simulink model "Ctrl_WT_openPI_delay"  (R2019b)
settings: Solver=ode23tb  StartTime=0.0  StopTime=30  MaxStep=1/60  RelTol=1e-4  AbsTol=1e-3  EnableMultiTasking=on
InitFcn:
  | xInitial = init_power_wind_ig;
libraries: cstblocks x7
settings Model: PauseTimes=15  ExtModeAutoUpdateStatusClock=off  Creator=MathWorks  LastModifiedBy=estuser04
settings SolverCC: AutoScaleAbsTol=off  SolverResetMethod=Robust
settings DataIOCC: LimitDataPoints=on  SaveFormat=Array  SignalLoggingSaveFormat=ModelDataLogs  SaveOutput=off  SaveTime=off  ReturnWorkspaceOutputs=off  SignalLoggingName=logsOut
settings OptimizationCC: BlockReduction=off  DefaultParameterBehavior=Inlined  BufferReuse=off  ExpressionDepthLimit=2147483647  InitFltsAndDblsToZero=on  LifeSpan=inf
settings DebuggingCC: UnderspecifiedInitializationDetection=Classic  MergeDetectMultiDrivingBlocksExec=none  CheckExecutionContextPreStartOutputMsg=on  CheckExecutionContextRuntimeOutputMsg=on  SignalResolutionControl=TryResolveAllWithWarning  SolverPrmCheckMsg=warning  MultiTaskDSMMsg=warning  MultiTaskCondExecSysMsg=none  FcnCallInpInsideContextMsg=warning  StateNameClashWarn=warning  InitInArrayFormatMsg=none  SFUnexpectedBacktrackingDiag=warning  SFNoUnconditionalDefaultTransitionDiag=warning  SFExecutionAtInitializationDiag=none  ArithmeticOperatorsInVariantConditions=warning
settings HardwareCC: ProdBitPerPointer=32  ProdBitPerSizeT=32  ProdBitPerPtrDiffT=32  ProdLargestAtomicFloat=None  ProdIntDivRoundTo=Undefined  ProdEndianess=Unspecified  ProdWordSize=32  ProdHWDeviceType=32-bit Generic
settings ModelReferenceCC: PropagateSignalLabelsOutOfModel=off
settings SFSimCC: SimUseLocalCustomCode=off  CustomCodeUndefinedFunction=UseInterfaceOnly
settings RTWCC: RTWUseLocalCustomCode=off
settings CodeAppCC: StateflowObjectComments=on
settings GRTTargetCC: TargetLangStandard=C89/C90 (ANSI)  GeneratePreprocessorConditionals=Disable all  CombineOutputUpdateFcns=off  GRTInterface=on
settings ConfigComp: CovMetricSettings=dw  CovHtmlReporting=on  CovSaveCumulativeToWorkspaceVar=on  CovSaveSingleToWorkspaceVar=on  CovExternalEMLEnable=off  CovSFcnEnable=off
settings SimscapeCC: SimscapeNormalizeSystem=off

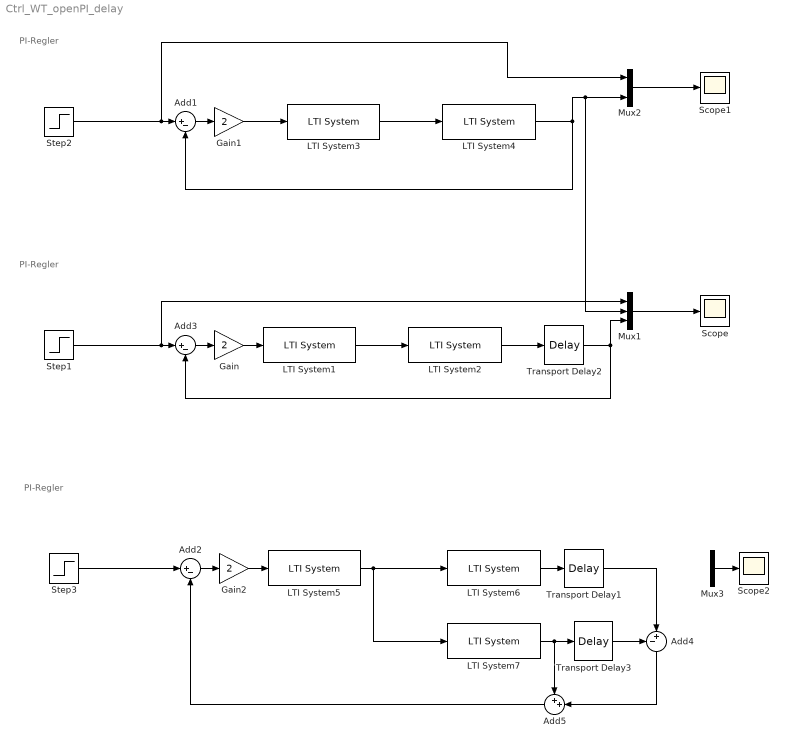
== system Ctrl_WT_openPI_delay ==
  note: PI-Regler
  note: PI-Regler
  note: PI-Regler
  Add1 : Sum  Inputs=|+-
  Add2 : Sum  Inputs=|+-
  Add3 : Sum  Inputs=|+-
  Add4 : Sum  Inputs=-+|
  Add5 : Sum  Inputs=++|
  Gain : Gain  Gain=2
  Gain1 : Gain  Gain=2
  Gain2 : Gain  Gain=2
  LTI System1 : cstblocks/LTI System  sys=GRegPI  IC=[]
  LTI System{2,4,6..7} (4 alike) : cstblocks/LTI System  sys=GProc  IC=[]
  LTI System3 : cstblocks/LTI System  sys=GRegPI  IC=[]
  LTI System5 : cstblocks/LTI System  sys=GRegPI  IC=[]
  Mux1 : Mux  Inputs=3
  Mux2 : Mux  Inputs=2
  Mux3 : Mux
  Scope : Scope
  Scope1 : Scope
  Scope2 : Scope
  Step1 : Step  Time=5  SampleTime=0
  Step2 : Step  Time=5  SampleTime=0
  Step3 : Step  Time=5  SampleTime=0
  Transport Delay1 : TransportDelay  DelayTime=1.1
  Transport Delay2 : TransportDelay  DelayTime=0.7
  Transport Delay3 : TransportDelay
  wires:
  Mux1/1 -> Scope/1
  Add3/1 -> Gain/1
  Step1/1 -> Add3/1, Mux1/1
  Gain/1 -> LTI System1/1
  LTI System1/1 -> LTI System2/1
  LTI System3/1 -> LTI System4/1
  Gain1/1 -> LTI System3/1
  Step2/1 -> Mux2/1, Add1/1
  Add1/1 -> Gain1/1
  Mux2/1 -> Scope1/1
  LTI System2/1 -> Transport Delay2/1
  Transport Delay2/1 -> Mux1/3, Add3/2
  LTI System6/1 -> Transport Delay1/1
  Gain2/1 -> LTI System5/1
  Step3/1 -> Add2/1
  Add2/1 -> Gain2/1
  LTI System7/1 -> Add5/1, Transport Delay3/1
  Transport Delay1/1 -> Add4/2
  Transport Delay3/1 -> Add4/1
  Add4/1 -> Add5/2
  Add5/1 -> Add2/2
  Mux3/1 -> Scope2/1
  LTI System5/1 -> LTI System6/1, LTI System7/1
  LTI System4/1 -> Add1/2, Mux1/2, Mux2/2
